simulink model "DSB_Modulation"  (R2019b)
settings: Solver=VariableStepAuto  StartTime=0.0  StopTime=40/15000  RelTol=1e-3
settings Model: Creator=Lenovo  LastModifiedBy=Lenovo

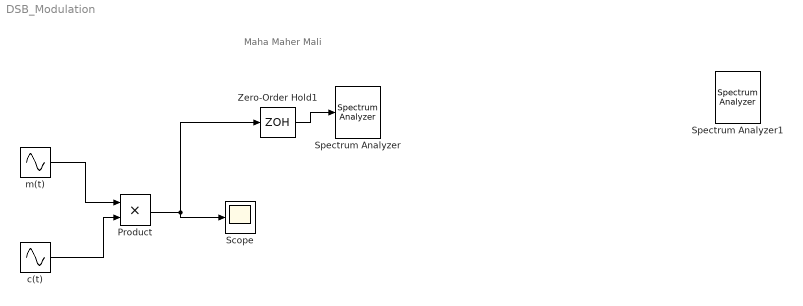
== system DSB_Modulation ==
  note: Maha Maher Mali
  Product : Product
  Scope : Scope
  Spectrum Analyzer : SpectrumAnalyzer
  Spectrum Analyzer1 : SpectrumAnalyzer
  Zero-Order Hold1 : ZeroOrderHold  SampleTime=1/(10*15e3)
  c(t) : Sin  Frequency=2*pi*15000  SampleTime=0
  m(t) : Sin  Amplitude=0.85  Frequency=2*pi*1000  SampleTime=0
  wires:
  m(t)/1 -> Product/1
  c(t)/1 -> Product/2
  Product/1 -> Zero-Order Hold1/1, Scope/1
  Zero-Order Hold1/1 -> Spectrum Analyzer/1
